simulink model "feedbackTuning"  (R2016b)
settings: Solver=VariableStepAuto  StartTime=0.0  StopTime=0.3  RelTol=1e-3
values from neighbouring files (symbols this model uses):
  denominator = denominator{1}    [mainFeedbackTuning.m]
  denRigidBody = den    [mainFeedbackTuning.m]
  m = 25    [mainFeedbackTuning.m]
  numerator = numerator{1}    [mainFeedbackTuning.m]
  numRigidBody = num    [mainFeedbackTuning.m]
  Ts = 1/fs    (= 0.0001)    [mainFeedbackTuning.m]
  varNoise = sigma*sigma    (= 1e-16)    [mainFeedbackTuning.m]
libraries: simulink x1, model_controller x1
settings Model: Creator=Dai Luyao  LastModifiedBy=Dai Luyao

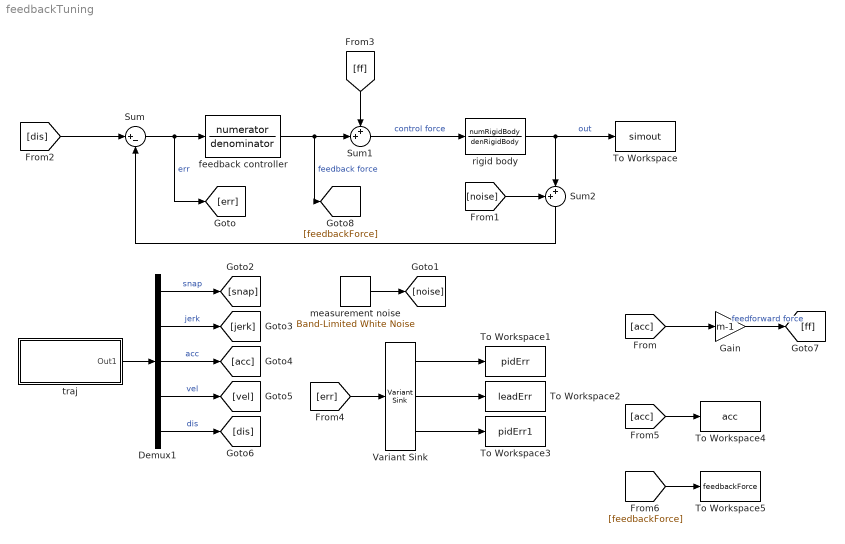
== system feedbackTuning ==
  Demux1 : Demux  Outputs=5
  Gain : Gain  Gain=m-1
  Sum : Sum  Inputs=|+-
  Sum1 : Sum  Inputs=++|
  Sum2 : Sum  Inputs=++|
  To Workspace : ToWorkspace  VariableName=simout  SampleTime=-1
  To Workspace1 : ToWorkspace  VariableName=pidErr  SaveFormat=Structure With Time  SampleTime=-1
  To Workspace2 : ToWorkspace  VariableName=leadErr  SaveFormat=Structure With Time  SampleTime=-1
  To Workspace3 : ToWorkspace  VariableName=pidErr1  SaveFormat=Structure With Time  SampleTime=-1
  To Workspace4 : ToWorkspace  VariableName=acc  SaveFormat=Structure With Time  SampleTime=-1
  To Workspace5 : ToWorkspace  VariableName=feedbackForce  SaveFormat=Structure With Time  SampleTime=-1
  Variant Sink : VariantSink
  feedback controller : TransferFcn  Numerator=numerator  Denominator=denominator
  measurement noise : simulink/Sources/Band-Limited White Noise  Cov=[varNoise*Ts]  Ts=Ts  seed=[23341]
  rigid body : TransferFcn  Numerator=numRigidBody  Denominator=denRigidBody
  traj : Subsystem  BlockChoice=4th order traj
      settings: AttributesFormatString=%<BlockChoice>  TemplateBlock=model_controller/Profile Generators/traj  MemberBlocks=2th order traj,3rd order traj,4th order traj,step
  wires:
  rigid body/1 -> Sum2/2, To Workspace/1  "out"
  Demux1/1 -> [snap]  "snap"
  Demux1/2 -> [jerk]  "jerk"
  Demux1/3 -> [acc]  "acc"
  Demux1/4 -> [vel]  "vel"
  Demux1/5 -> [dis]  "dis"
  feedback controller/1 -> [feedbackForce], Sum1/2  "feedback force"
  Sum/1 -> [err], feedback controller/1  "err"
  [acc] -> Gain/1
  traj/1(Out1) -> Demux1/1
  measurement noise/1 -> [noise]
  [noise] -> Sum2/1
  [err] -> Variant Sink/1
  Variant Sink/1 -> To Workspace1/1
  Variant Sink/2 -> To Workspace2/1
  Variant Sink/3 -> To Workspace3/1
  Sum1/1 -> rigid body/1  "control force"
  Sum2/1 -> Sum/2
  [dis] -> Sum/1
  Gain/1 -> [ff]  "feedforward force"
  [acc] -> To Workspace4/1
  [feedbackForce] -> To Workspace5/1
  [ff] -> Sum1/1

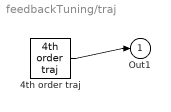
== system feedbackTuning/traj ==
  4th order traj : model_controller/Profile Generators/4th order traj  t0=0  x=0.06  v=0.25  a=10  j=800  d=64000  Ts=0
  Out1 : Outport
  wires:
  4th order traj/1 -> Out1/1
